simulink model "pwm2"  (R2012b)
settings: Solver=ode45  StartTime=0.0  StopTime=0.5  FixedStep=0.4e-4  MaxStep=1e-5  RelTol=1e-3
libraries: BLDC x2, Tools x1
settings Model: Creator=h3now  LastModifiedBy=h3now

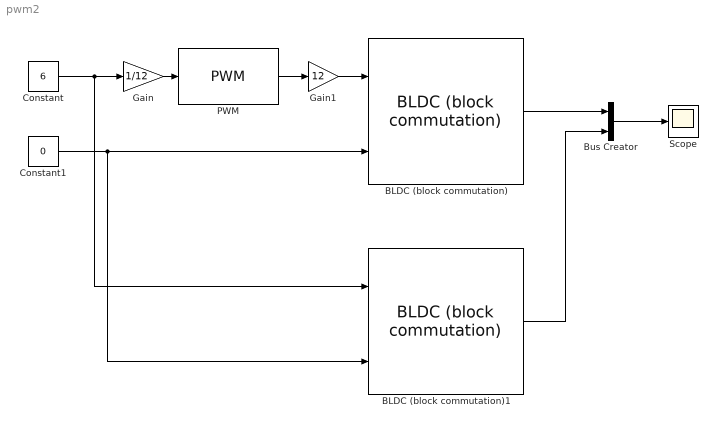
== system pwm2 ==
  BLDC (block commutation) : BLDC/BLDC (block commutation)  J=1.39e-6  R=10.1/2  L=2.04/2000  P=8  Kt=15.7e-3/1.19  Ke=15.7e-3/1.19  Kd=0
  BLDC (block commutation)1 : BLDC/BLDC (block commutation)  J=1.39e-6  R=10.1/2  L=2.04/2000  P=8  Kt=15.7e-3/1.19  Ke=15.7e-3/1.19  Kd=0
  Bus Creator : BusCreator  Inputs=2
  Constant : Constant  Value=6
  Constant1 : Constant  Value=0
  Gain : Gain  Gain=1/12
  Gain1 : Gain  Gain=12
  PWM : Tools/PWM  f=10000
  Scope : Scope
  wires:
  PWM/1 -> Gain1/1
  Gain/1 -> PWM/1
  Constant/1 -> BLDC (block commutation)1/1, Gain/1
  Gain1/1 -> BLDC (block commutation)/1
  BLDC (block commutation)/2 -> Bus Creator/1
  BLDC (block commutation)1/2 -> Bus Creator/2
  Bus Creator/1 -> Scope/1
  Constant1/1 -> BLDC (block commutation)1/2, BLDC (block commutation)/2
